simulink model "Stewart3"  (R2016a)
settings: Solver=FixedStepAuto  StartTime=0.0  StopTime=inf  RelTol=1e-3
settings Model: ExtModeTrigDuration=2  Creator=costa  LastModifiedBy=costa
settings OptimizationCC: OptimizeModelRefInitCode=on  LifeSpan=1  MaxStackSize=64
settings HardwareCC: ProdBitPerInt=16  ProdBitPerPointer=16  ProdLargestAtomicFloat=None  ProdWordSize=8  ProdHWDeviceType=Atmel->AVR
settings RTWCC: SystemTargetFile=ert.tlc  HardwareBoard=Arduino Mega 2560  TemplateMakefile=ert_default_tmf  GenerateReport=on  Toolchain=Arduino AVR v1.6.1  BuildConfiguration=Faster Runs  IncludeHyperlinkInReport=on  LaunchReport=on  GenerateTraceInfo=on  GenerateTraceReport=on  GenerateTraceReportSl=on  GenerateTraceReportSf=on  GenerateTraceReportEml=on
settings CodeAppCC: ForceParamTrailComments=on  IgnoreCustomStorageClasses=off  OperatorAnnotations=on  SimulinkDataObjDesc=on  SFDataObjDesc=on  MATLABFcnDesc=on  MangleLength=10  InsertBlockDesc=on  MATLABSourceComments=on
settings ERTTargetCC: SupportContinuousTime=on  SupportVariableSizeSignals=on  ExtMode=on  ExtModeTransport=3  ExtModeMexFile=ext_serial_win32_comm_rtt  ExtModeMexArgs=0 5 115200

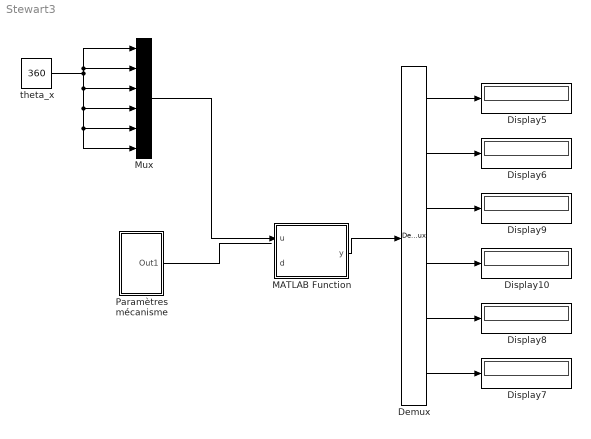
== system Stewart3 ==
  Demux : Demux  Outputs=6
  Display{5..10} (6 alike) : Display
  MATLAB Function : MATLAB Function  TreatAsAtomicUnit=on
  Mux : Mux  Inputs=6
  Paramètres mécanisme : Subsystem
  theta_x : Constant  Value=360
  wires:
  Mux/1 -> MATLAB Function/1(u)
  MATLAB Function/1(y) -> Demux/1
  Demux/1 -> Display5/1
  Demux/2 -> Display6/1
  Demux/3 -> Display9/1
  Demux/4 -> Display10/1
  Demux/5 -> Display8/1
  Demux/6 -> Display7/1
  theta_x/1 -> Mux/2, Mux/1, Mux/6, Mux/5, Mux/4, Mux/3
  Paramètres mécanisme/1(Out1) -> ?

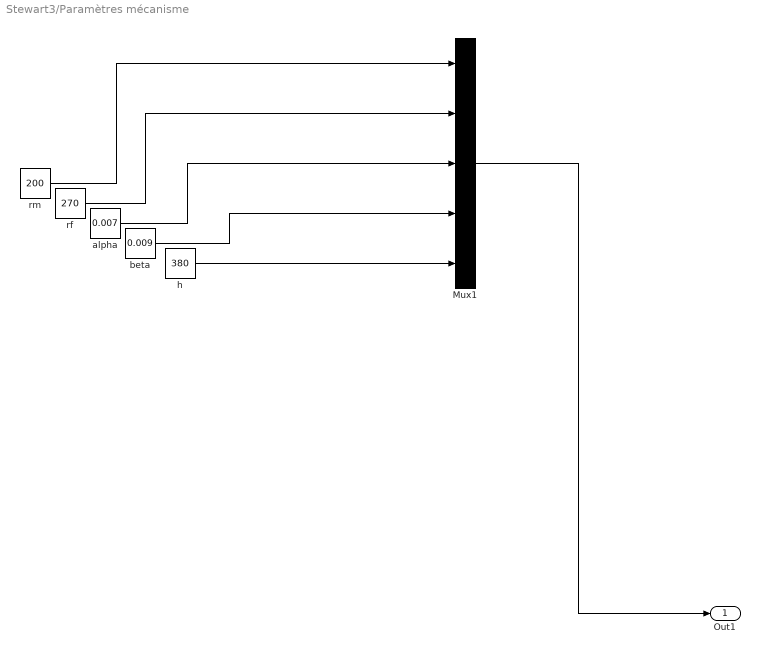
== system Stewart3/Paramètres mécanisme ==
  Mux1 : Mux  Inputs=5
  alpha : Constant  Value=0.007
  beta : Constant  Value=0.009
  h : Constant  Value=380
  rf : Constant  Value=270
  rm : Constant  Value=200
  Out1 : Outport
  wires:
  Mux1/1 -> Out1/1
  rm/1 -> Mux1/1
  rf/1 -> Mux1/2
  alpha/1 -> Mux1/3
  beta/1 -> Mux1/4
  h/1 -> Mux1/5

== matlab function Stewart3/MATLAB Function ==
  data: u input size=6; y output size=5; d input
function y = fcn(u,d)
%#codegen
x0=[0,0,0,0,0,0];
coder.extrinsic('myFunc')
y = myFunc(u,d,x0);
